simulink model "abastecimento_simulacao"  (R2018a)
settings: Solver=VariableStepAuto  StartTime=0.0  StopTime=100000  RelTol=1e-3
libraries: sh_lib x7, fl_lib x4, nesl_utility x3
settings Model: Creator=dougl  LastModifiedBy=LUISA

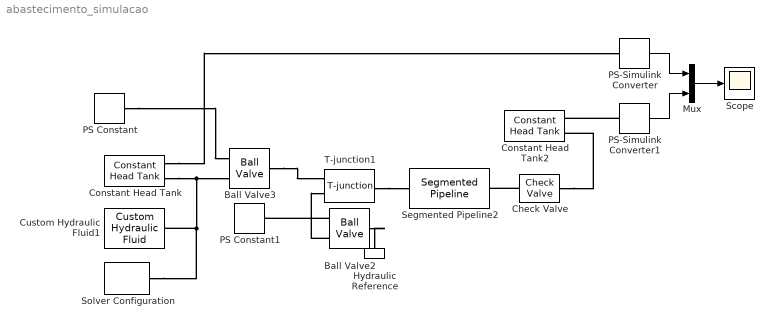
== system abastecimento_simulacao ==
  Ball Valve2 : sh_lib/Valves/Flow Control Valves/Ball Valve  valve_seat_spec=1  cone_ang=120 deg  d_ball=15 mm  d_orif=15.8 mm  x_0=0 mm  C_d=0.65  A_leak=1e-12 m^2  lam_spec=1  B_lam=0.999  Re_cr=10  flow_rate_specify=on  flow_rate_priority=High  flow_rate=12.7 m^3/s  flow_rate_nominal_specify=off  flow_rate_nominal_unit=m^3/s  flow_rate_nominal_value=1  pressure_drop_specify=off  pressure_drop_priority=None  pressure_drop=0 Pa  pressure_drop_nominal_specify=off  pressure_drop_nominal_unit=Pa  pressure_drop_nominal_value=1
      settings: SourceProductName=Simscape Fluids  SourceProductBaseCode=SH  LogSimulationData=on
  Ball Valve3 : sh_lib/Valves/Flow Control Valves/Ball Valve  valve_seat_spec=1  cone_ang=120 deg  d_ball=15 mm  d_orif=15.8 mm  x_0=0 mm  C_d=0.65  A_leak=1e-12 m^2  lam_spec=1  B_lam=0.999  Re_cr=10  flow_rate_specify=on  flow_rate_priority=High  flow_rate=12.7 m^3/s  flow_rate_nominal_specify=off  flow_rate_nominal_unit=m^3/s  flow_rate_nominal_value=1  pressure_drop_specify=off  pressure_drop_priority=None  pressure_drop=0 Pa  pressure_drop_nominal_specify=off  pressure_drop_nominal_unit=Pa  pressure_drop_nominal_value=1
      settings: SourceProductName=Simscape Fluids  SourceProductBaseCode=SH  LogSimulationData=on
  Check Valve : sh_lib/Valves/Directional Valves/Check Valve  area_max=1e-4 m^2  pres_crack=0.3e5 Pa  pres_max=1.2e5 Pa  C_d=0.7  A_leak=1e-12 m^2  lam_spec=1  B_lam=0.999  Re_cr=12  dynamic=0  tau=0.1 s  area_init=1e-12 m^2
      settings: SourceProductName=Simscape Fluids  SourceProductBaseCode=SH
  Constant Head Tank : sh_lib/Low-Pressure Blocks/Constant Head Tank  press=57 Pa  fluid_level=1 m  pipe_diam=0.02 m  loss_coeff=1.2  g=9.80665 m/s^2  volume_specify=on  volume_priority=High  volume=7 l  volume_nominal_specify=off  volume_nominal_unit=m^3  volume_nominal_value=1
      settings: SourceProductName=Simscape Fluids  SourceProductBaseCode=SH
  Constant Head Tank2 : sh_lib/Low-Pressure Blocks/Constant Head Tank  press=30 Pa  fluid_level=0 m  pipe_diam=0.02 m  loss_coeff=1.2  g=9.80665 m/s^2  volume_specify=on  volume_priority=High  volume=0 l  volume_nominal_specify=off  volume_nominal_unit=m^3  volume_nominal_value=1
      settings: SourceProductName=Simscape Fluids  SourceProductBaseCode=SH
  Custom Hydraulic Fluid1 : fl_lib/Hydraulic/Hydraulic Utilities/Custom Hydraulic Fluid  density=750 kg/m^3  viscosity_kin=0.0639e-6 m^2/s  bulk=0.8e9 Pa  alpha=0  range_error=2
      settings: SourceProductName=Simscape  SourceProductBaseCode=SS
  Hydraulic Reference : fl_lib/Hydraulic/Hydraulic Elements/Hydraulic Reference
      settings: SourceProductName=Simscape
  Mux : Mux  Inputs=2
  PS Constant : fl_lib/Physical Signals/Sources/PS Constant  constant=0.019
  PS Constant1 : fl_lib/Physical Signals/Sources/PS Constant  constant=0
  PS-Simulink Converter : nesl_utility/PS-Simulink Converter  PhysicalDomain=network_engine_domain  SubClassName=ps_output  LeftPortType=input  RightPortType=output  PseudoPeriodic=off  Frequencies=[]  Unit=l  AffineConversion=off
  PS-Simulink Converter1 : nesl_utility/PS-Simulink Converter  PhysicalDomain=network_engine_domain  SubClassName=ps_output  LeftPortType=input  RightPortType=output  PseudoPeriodic=off  Frequencies=[]  Unit=l  AffineConversion=off
  Scope : Scope
  Segmented Pipeline2 : sh_lib/Pipelines/Segmented Pipeline  d_in=0.01 m  length=5 m  segm_num=1  length_ad=1 m  roughness=1.5e-5 m  Re_lam=2e+3  Re_turb=4e+3  wall_type=1  pr_r_coef=2e-10 m/Pa  time_const=0.008 s  k_sh=1.4  init_pr_option=1  initial_pressure=0 Pa  initial_pressure_vector=0 Pa  initial_flow_rate=0 m^3/s
      settings: SourceProductName=Simscape Fluids  SourceProductBaseCode=SH
  Solver Configuration : nesl_utility/Solver Configuration  PhysicalDomain=network_engine_domain  SubClassName=solver  LeftPortType=input  RightPortType=generic  Tones=[]  Harmonics=[]  SimulateNoise=off  Profile=off  UseLocalSampling=off  EnableSwitchedLinearOptims=on  FrequencyDomain=off  UseCCode=off  RelTol=0.001  AbsTol=1e-06  MinStep=1e-09  ToWorkspace=off  RevertToSquareIcSolve=off  NumHomotopyIterations=100  PhasorMode=off  PhasorModeNumHarmonics=1  DoDC=off  ResidualTolerance=1e-09  UseLocalSolver=off  LocalSolverChoice=NE_BACKWARD_EULER_ADVANCER  LocalSolverSampleTime=0.001  DoFixedCost=off  MaxNonlinIter=3  MaxModeIter=2  LinearAlgebra=Sparse  EquationFormulation=NE_TIME_EF  DelaysMemoryBudget=1024  AutomaticFiltering=on  FilteringTimeConstant=0.001
  T-junction1 : sh_lib/Local Hydraulic Resistances/T-junction  main_diam=0.01 m  branch_diam=0.01 m  kp_ab=1  kp_ba=1  kp_aa1=1  kp_a1a=1  kp_a1b=1  kp_ba1=1  lam_spec=1  B_lam=0.999  Re_cr=120
      settings: SourceProductName=Simscape Fluids  SourceProductBaseCode=SH
  wires:
  Mux/1 -> Scope/1
  PS-Simulink Converter/1 -> Mux/1
  PS-Simulink Converter1/1 -> Mux/2
  connections:
  Constant Head Tank/RConn2 -- Ball Valve3/LConn2 -- Solver Configuration/RConn1 -- Custom Hydraulic Fluid1/RConn1
  Ball Valve2/LConn2 -- T-junction1/LConn2
  Ball Valve3/RConn1 -- T-junction1/LConn1
  T-junction1/RConn1 -- Segmented Pipeline2/LConn1
  Check Valve/LConn1 -- Segmented Pipeline2/RConn1
  Check Valve/RConn1 -- Constant Head Tank2/RConn2
  PS-Simulink Converter1/LConn1 -- Constant Head Tank2/RConn1
  Ball Valve2/RConn1 -- Hydraulic Reference/LConn1
  Constant Head Tank/RConn1 -- PS-Simulink Converter/LConn1
  PS Constant/RConn1 -- Ball Valve3/LConn1
  Ball Valve2/LConn1 -- PS Constant1/RConn1
